simulink model "wlan_phy_tx_pmd"  (Simulink 7.8)
settings: Solver=VariableStepDiscrete  SolverMode=SingleTasking  StartTime=0.0  StopTime=inf  RelTol=1e-3
PostLoadFcn:
  | wlan_phy_tx_init
InitFcn:
  | wlan_phy_tx_init
StartFcn:
  | wlan_phy_tx_init
undefined symbols (not defined in the file): gcbh, ht_preamble_rom, MAX_CP_LEN, MAX_DATA_BITS_PER_SYM_PERIOD, MAX_NCBPS, MAX_NUM_BYTES, MAX_NUM_SC, MAX_NUM_SYMS, mcs_rom_11ag, mcs_rom_11n, Mod_Constellation_16QAM, Mod_Constellation_64QAM, Mod_Constellation_BPSK, Mod_Constellation_QPSK, Preamble_IQ, Preamble_IQ_scaled, tx_sim, wlan_tx_interleave_rom, xlBlockLoadCallback, xlGetNormalizedPeriod
libraries: xbsIndex_r4 x1358, xbsEDKLib_r4 x1
(part 3 of 10)

== system wlan_phy_tx_pmd/HT Preamble Gen ==
  Sym Cfg : Inport
  Start : Inport  Port=2
  IQ FIFO tready : Inport  Port=3
  Bus Creator : BusCreator
  Concat : xbsIndex_r4/Concat  num_inputs=2  dbl_ovrd=off  block_type=concat
  Constant9 : xbsIndex_r4/Constant  const=ceil(length(ht_preamble_rom)/2) - 1  gui_display_data_type=Fixed-point  arith_type=Unsigned  n_bits=ceil(log2(length(ht_preamble_rom)))-1  bin_pt=0  preci_type=Single  exp_width=8  frac_width=24  explicit_period=off  period=1  equ=P=C  opselect=C  inp2=PCIN>>17  opr=+  inp1=P  carry=CIN  dbl_ovrd=off  block_type=constant
  Counter1 : xbsIndex_r4/Counter  cnt_type=Free Running  cnt_to=Inf  operation=Up  start_count=0  cnt_by_val=1  arith_type=Unsigned  n_bits=ceil(log2(length(ht_preamble_rom)))-1  bin_pt=0  load_pin=off  rst=on  en=on  explicit_period=off  period=1  dbl_ovrd=off  use_behavioral_HDL=off  implementation=Fabric  block_type=counter
  Delay{,1..3} (4 alike) : xbsIndex_r4/Delay  rst=off  infoeditControl=Selection of Reset will increase slice count due to use of real FFs and instead of SRLs  en=off  latency=1  dbl_ovrd=off  reg_retiming=off  block_type=delay
  HT Training I : xbsIndex_r4/ROM  depth=length(ht_preamble_rom)  initVector=real(ht_preamble_rom)  distributed_mem=Distributed memory  rst=off  init_reg=0  en=off  latency=1  gui_display_data_type=Fixed-point  arith_type="Signed  (2's comp)"  n_bits=16  bin_pt=15  preci_type=Single  exp_width=8  frac_width=24  dbl_ovrd=off  optimize=Area  use_rpm=on  block_type=sprom
  HT Training Q : xbsIndex_r4/ROM  depth=length(ht_preamble_rom)  initVector=imag(ht_preamble_rom)  distributed_mem=Distributed memory  rst=off  init_reg=0  en=off  latency=1  gui_display_data_type=Fixed-point  arith_type="Signed  (2's comp)"  n_bits=16  bin_pt=15  preci_type=Single  exp_width=8  frac_width=24  dbl_ovrd=off  optimize=Area  use_rpm=on  block_type=sprom
  Inverter1 : xbsIndex_r4/Inverter  en=off  latency=0  dbl_ovrd=off  block_type=inv
      settings: xl_area=[0 0 0 0 0 0 0]  block_version=VER_STRING_GOES_HERE
  Logical1 : xbsIndex_r4/Logical  logical_function=OR  inputs=2  en=off  latency=0  precision=Full  arith_type=Unsigned  n_bits=8  bin_pt=2  align_bp=on  dbl_ovrd=off  block_type=logical
      settings: xl_area=[1 0 0 1 0 0 0]  block_version=VER_STRING_GOES_HERE
  Logical2 : xbsIndex_r4/Logical  logical_function=OR  inputs=2  en=off  latency=0  precision=Full  arith_type=Unsigned  n_bits=8  bin_pt=2  align_bp=on  dbl_ovrd=off  block_type=logical
      settings: xl_area=[1 0 0 1 0 0 0]  block_version=VER_STRING_GOES_HERE
  Logical3 : xbsIndex_r4/Logical  logical_function=AND  inputs=2  en=off  latency=0  precision=Full  arith_type=Unsigned  n_bits=8  bin_pt=2  align_bp=on  dbl_ovrd=off  block_type=logical
      settings: xl_area=[1 0 0 1 0 0 0]  block_version=VER_STRING_GOES_HERE
  Logical4 : xbsIndex_r4/Logical  logical_function=AND  inputs=2  en=off  latency=0  precision=Full  arith_type=Unsigned  n_bits=8  bin_pt=2  align_bp=on  dbl_ovrd=off  block_type=logical
      settings: xl_area=[1 0 0 1 0 0 0]  block_version=VER_STRING_GOES_HERE
  MCode : xbsIndex_r4/MCode  mfname=sym_config_decode  explicit_period=on  period=1  inputsTable={'boundInpExpr'=>[''],'inputs'=>['sym_cfg']}  outputsTable={'outputs'=>['load_base_rate','rotate_bpsk','load_htstf','load_htltf','load_full_rate','pilot_shift','cyclic_prefix','cyclic_shift'],'suppressOut'=>['off','off','off','off','off','off','off','off']}  dbl_ovrd=off  enable_stdout=off  enable_debug=off  suppress_output=on  defparams={}  hide_port_list={}  block_type=mcode
  Relational2 : xbsIndex_r4/Relational  mode=a>=b  en=off  latency=0  dbl_ovrd=off  block_type=relational
  S-R Latch1 : Subsystem
  " Sym Cfg" : Outport
  IQ stream : Outport  Port=2
  wires:
  Counter1/1 -> Concat/2, Relational2/1
  Constant9/1 -> Relational2/2
  Inverter1/1 -> Counter1/1
  S-R Latch1/1(Q) -> Inverter1/1, Delay1/1, Logical4/1
  [TX_RESET] -> Logical2/1
  Relational2/1 -> Logical2/2, Delay2/1
  Logical2/1 -> S-R Latch1/2(R)
  Concat/1 -> HT Training I/1, HT Training Q/1
  MCode/4 -> Logical1/1, Delay3/1
  HT Training I/1 -> Bus Creator/1  "I"
  HT Training Q/1 -> Bus Creator/2  "Q"
  Logical3/1 -> S-R Latch1/1(S)
  Start/1 -> Logical3/2
  Sym Cfg/1 -> Delay/1, MCode/1
  MCode/3 -> Logical1/2
  Logical1/1 -> Logical3/1
  Delay/1 -> " Sym Cfg"/1
  Delay1/1 -> Bus Creator/3  "IQ tvalid"
  Delay2/1 -> Bus Creator/4  "IQ tlast"
  Bus Creator/1 -> IQ stream/1
  Logical4/1 -> Counter1/2
  IQ FIFO tready/1 -> Logical4/2
  Delay3/1 -> Concat/1

== system wlan_phy_tx_pmd/IFFT and Cyclic Prefix ==
  Sym Cfg : Inport
  I : Inport  Port=2
  Q : Inport  Port=3
  IQ Valid : Inport  Port=4
  IQ tlast : Inport  Port=5
  Buffer and Cyclic Prefix : Subsystem
  FFT Core : Subsystem
  FIFO : Subsystem
  " I" : Outport
  " Q" : Outport  Port=2
  " IQ Valid" : Outport  Port=3
  FIFO tready : Outport  Port=4
  wires:
  FFT Core/2(I out) -> Buffer and Cyclic Prefix/1(I)
  FFT Core/3(Q out) -> Buffer and Cyclic Prefix/2(Q)
  FFT Core/4(data_xk_index) -> Buffer and Cyclic Prefix/3(xkindex)
  FFT Core/5(data_out_tvalid) -> Buffer and Cyclic Prefix/4(tvalid)
  FFT Core/6(data_out_tlast) -> Buffer and Cyclic Prefix/5(tlast)
  FFT Core/1(data_in_tready) -> FIFO/1(FFT tready)
  FIFO/1(" I") -> FFT Core/1("I ")
  Buffer and Cyclic Prefix/1(" I") -> " I"/1
  Buffer and Cyclic Prefix/2(" Q") -> " Q"/1
  FIFO/3(" IQ tvalid") -> FFT Core/3(IQ In Valid)
  Buffer and Cyclic Prefix/3(" valid") -> " IQ Valid"/1
  FIFO/4(IQ tlast) -> FFT Core/4(IQ tlast)
  FIFO/5(Sym cfg) -> Buffer and Cyclic Prefix/6(Sym Cfg)
  Sym Cfg/1 -> FIFO/2(Sym Cfg)
  I/1 -> FIFO/3(I)
  Q/1 -> FIFO/4(Q)
  IQ Valid/1 -> FIFO/5(IQ tvalid)
  IQ tlast/1 -> FIFO/6("IQ tlast ")
  FIFO/2(" Q") -> FFT Core/2("Q ")
  FIFO/6(FIFO tready) -> FIFO tready/1

== system wlan_phy_tx_pmd/Mux ==
  Preamble Sym Cfg : Inport
  Preamble IQ : Inport  Port=2
  PSDU Sym Cfg : Inport  Port=3
  PSDU IQ : Inport  Port=4
  Bus Selector : BusSelector  OutputSignals=I,Q,IQ tvalid,IQ tlast
  Bus Selector1 : BusSelector  OutputSignals=I,Q,IQ tvalid,IQ tlast
  Mux{1..4,6} (5 alike) : xbsIndex_r4/Mux  inputs=2  en=off  latency=0  precision=Full  arith_type=Unsigned  n_bits=16  bin_pt=14  quantization=Truncate  overflow=Wrap  dbl_ovrd=off  block_type=mux
  Sym Cfg : Outport
  " I" : Outport  Port=2
  " Q" : Outport  Port=3
  " IQ tvalid" : Outport  Port=4
  IQ tlast : Outport  Port=5
  wires:
  Mux6/1 -> " I"/1
  Mux1/1 -> " Q"/1
  Mux2/1 -> " IQ tvalid"/1
  Mux3/1 -> IQ tlast/1
  Preamble IQ/1 -> Bus Selector/1
  Bus Selector/1 -> Mux6/2  "<I>"
  Bus Selector/2 -> Mux1/2  "<Q>"
  Bus Selector/3 -> Mux2/2  "<IQ tvalid>"
  Bus Selector/4 -> Mux3/2  "<IQ tlast>"
  PSDU IQ/1 -> Bus Selector1/1
  Bus Selector1/4 -> Mux3/3  "<IQ tlast>"
  Bus Selector1/1 -> Mux6/3  "<I>"
  Bus Selector1/2 -> Mux1/3  "<Q>"
  Bus Selector1/3 -> Mux2/1, Mux1/1, Mux6/1, Mux2/3, Mux3/1, Mux4/1  "<IQ tvalid>"
  PSDU Sym Cfg/1 -> Mux4/3
  Preamble Sym Cfg/1 -> Mux4/2
  Mux4/1 -> Sym Cfg/1

== system wlan_phy_tx_pmd/OFDM Symbol Ctrl ==
  note: Stop generating symbols after DATA field is complete
  note: Stop generating symbols if TX_RESET asserts early
  note: This block generates two outputs:
      | Start Sym: triggers generation of one OFDM symbol from the Tx pipeline
      | Sym Cfg: parameters required to generate the new OFDM symbol
      |
      | Timing of Start Sym is critical:
      | Immediately after "Start Tx" this block triggers computation of 3 OFDM symbols. The resulting
      | samples are stored in the FIFO in the "Outputs" block. Samples will be read from this FIFO after
      | the preamble. Once the FIFO occupancy drops below 180 samples (first 3 symbols occupy 240
      | samples), the next OFDM symbol is started. From this point forward a new OFDM symbol is
      | started every N sample periods, where N is the number of samples in the previous OFDM symbol
      | (N = num_subcarriers + cyclic_prefix_length). This timing ensures the output FIFO always has
      | enough samples to sustain a constant stream to the DACs, while adapting to changes in the
      | sampling rate and number of samples in each OFDM symbol / cyclic prefix.
      |
      | The Start Sym signal stops asserting after the final OFDM symbol is computed, indicated by the
      | DATA field being complete.
      |
      | The selection of the 180 sample threshold above is critical. A higher threshold will overflow the FIFO
      | with low MCS and low Tx sample rate. A lower thrshold will underflow the FIFO for high MCS and high
      | sample rate. This threshold will need tweaking for any big changes in Tx pipeline latency.
  Start Tx : Inport
  Sym Done : Inport  Port=2
  Data Done : Inport  Port=3
  Constant1 : xbsIndex_r4/Constant  const=180  gui_display_data_type=Fixed-point  arith_type=Unsigned  n_bits=8  bin_pt=0  preci_type=Single  exp_width=8  frac_width=24  explicit_period=off  period=1  equ=P=C  opselect=C  inp2=PCIN>>17  opr=+  inp1=P  carry=CIN  dbl_ovrd=off  block_type=constant
  Constant2 : xbsIndex_r4/Constant  const=2  gui_display_data_type=Fixed-point  arith_type=Unsigned  n_bits=2  bin_pt=0  preci_type=Single  exp_width=8  frac_width=24  explicit_period=off  period=1  equ=P=C  opselect=C  inp2=PCIN>>17  opr=+  inp1=P  carry=CIN  dbl_ovrd=off  block_type=constant
  Constant4 : xbsIndex_r4/Constant  const=20  gui_display_data_type=Fixed-point  arith_type=Unsigned  n_bits=5  bin_pt=0  preci_type=Single  exp_width=8  frac_width=24  explicit_period=off  period=1  equ=P=C  opselect=C  inp2=PCIN>>17  opr=+  inp1=P  carry=CIN  dbl_ovrd=off  block_type=constant
  Gateway Out{1..6,10} (7 alike) : xbsIndex_r4/Gateway Out  inherit_from_input=off  hdl_port=off  timing_constraint=None  locs_specified=off  LOCs={}  UseAsDAC=off  DACChannel='1'  block_type=gatewayout
  Inverter1 : xbsIndex_r4/Inverter  en=off  latency=0  dbl_ovrd=off  block_type=inv
  Inverter2 : xbsIndex_r4/Inverter  en=off  latency=0  dbl_ovrd=off  block_type=inv
  Logical1 : xbsIndex_r4/Logical  logical_function=AND  inputs=2  en=off  latency=0  precision=Full  arith_type=Unsigned  n_bits=8  bin_pt=2  align_bp=on  dbl_ovrd=off  block_type=logical
      settings: xl_area=[1 0 0 1 0 0 0]  block_version=VER_STRING_GOES_HERE
  Logical2 : xbsIndex_r4/Logical  logical_function=OR  inputs=4  en=off  latency=0  precision=Full  arith_type=Unsigned  n_bits=8  bin_pt=2  align_bp=on  dbl_ovrd=off  block_type=logical
      settings: xl_area=[1 0 0 1 0 0 0]  block_version=VER_STRING_GOES_HERE
  Logical3 : xbsIndex_r4/Logical  logical_function=AND  inputs=2  en=off  latency=0  precision=Full  arith_type=Unsigned  n_bits=8  bin_pt=2  align_bp=on  dbl_ovrd=off  block_type=logical
      settings: xl_area=[1 0 0 1 0 0 0]  block_version=VER_STRING_GOES_HERE
  Logical4 : xbsIndex_r4/Logical  logical_function=AND  inputs=3  en=off  latency=0  precision=Full  arith_type=Unsigned  n_bits=8  bin_pt=2  align_bp=on  dbl_ovrd=off  block_type=logical
      settings: xl_area=[1 0 0 1 0 0 0]  block_version=VER_STRING_GOES_HERE
  Logical5 : xbsIndex_r4/Logical  logical_function=AND  inputs=2  en=off  latency=0  precision=Full  arith_type=Unsigned  n_bits=8  bin_pt=2  align_bp=on  dbl_ovrd=off  block_type=logical
      settings: xl_area=[1 0 0 1 0 0 0]  block_version=VER_STRING_GOES_HERE
  Posedge1 : Subsystem
  Posedge2 : Subsystem
  Posedge3 : Subsystem
  Relational1 : xbsIndex_r4/Relational  mode=a<b  en=off  latency=0  dbl_ovrd=off  block_type=relational
  Relational2 : xbsIndex_r4/Relational  mode=a<=b  en=off  latency=0  dbl_ovrd=off  block_type=relational
  S-R Latch1 : Subsystem
  S-R Latch2 : Subsystem
  S-R Latch3 : Subsystem
  Slice : xbsIndex_r4/Slice  nbits=5  boolean_output=off  mode=Lower Bit Location + Width  bit1=0  base1=MSB of Input  bit0=0  base0=LSB of Input  dbl_ovrd=off  block_type=slice
  Sym Config Encode : Subsystem
  Sym Counter : Subsystem
  Sym Samp Counter : Subsystem
  Sym Start Ctrl : Scope  NumInputPorts=7
      settings: TimeRange=20000  YMin=0~0~0~0~0~0~0  YMax=1~1~1~1~250~7~16  SaveName=ScopeData3
  Sym Cfg : Outport
  " Start Sym" : Outport  Port=2
  wires:
  Sym Config Encode/1(Sym Cfg) -> Sym Cfg/1, Sym Samp Counter/2(Sym Cfg), Slice/1
  Sym Counter/1(Sym Ind) -> Relational1/1, Sym Config Encode/1(OFDM Sym Ind), Gateway Out6/1
  Gateway Out10/1 -> Sym Start Ctrl/3  "Sym Start"
  Gateway Out5/1 -> Sym Start Ctrl/4  "Sym Done"
  [OUTPUT_FIFO_OCC] -> Gateway Out1/1
  Gateway Out1/1 -> Sym Start Ctrl/5  "DAC FIFO Occ"
  Constant2/1 -> Relational1/2
  Start Tx/1 -> Posedge1/1(D)
  Sym Counter/2(" Start Sym") -> Logical4/1
  Posedge1/1(Q) -> Logical2/1, Gateway Out2/1, S-R Latch2/1(S)
  Sym Done/1 -> Gateway Out5/1, Logical3/2
  Relational1/1 -> Logical3/1
  Logical3/1 -> Logical2/2
  [OUTPUT_FIFO_OCC] -> Relational2/1
  Relational2/1 -> Posedge2/1(D)
  Constant1/1 -> Relational2/2
  Gateway Out2/1 -> Sym Start Ctrl/1  "Tx Start"
  Gateway Out3/1 -> Sym Start Ctrl/2  "Data Done"
  Gateway Out4/1 -> Sym Start Ctrl/7  "Sym Cfg"
  Gateway Out6/1 -> Sym Start Ctrl/6  "Sym Index"
  S-R Latch3/1(Q) -> Logical1/1, Inverter2/1
  Posedge3/1(Q) -> S-R Latch1/1(S), Gateway Out3/1
  Data Done/1 -> Posedge3/1(D)
  S-R Latch1/1(Q) -> Inverter1/1
  Logical4/1 -> " Start Sym"/1, Sym Samp Counter/1(Sym Started), Gateway Out10/1
  Inverter1/1 -> Logical4/2
  S-R Latch2/1(Q) -> Logical4/3
  Logical2/1 -> Sym Counter/1(Start Sym)
  Posedge2/1(Q) -> S-R Latch3/1(S), Logical5/1
  Sym Samp Counter/1(Start Next) -> Logical1/2
  Logical1/1 -> Logical2/4
  [TX_RESET] -> S-R Latch2/2(R), S-R Latch3/2(R), S-R Latch1/2(R)
  Slice/1 -> Gateway Out4/1
  Logical5/1 -> Logical2/3
  Inverter2/1 -> Logical5/2

== system wlan_phy_tx_pmd/PSDU Syms Gen ==
  note: This block implements the actual Tx PHY pipeline, from data bits to I/Q samples.
  Sym Cfg : Inport
  Start Sym : Inport  Port=2
  IQ FIFO tready : Inport  Port=3
  Bus Creator : BusCreator
  Convolutional Encoder : Subsystem
  Index Gen : Subsystem
  Modulate : Subsystem
  Pkt Data : Subsystem
  Puncture & Interleave : Subsystem
  " Sym Cfg" : Outport
  IQ stream : Outport  Port=2
  DATA Done : Outport  Port=3
  wires:
  Start Sym/1 -> Index Gen/2(Start Sym)
  Sym Cfg/1 -> Index Gen/1(Sym Cfg)
  Index Gen/1(" Sym Cfg") -> Pkt Data/1(Sym Cfg)
  Index Gen/2(Byte Ind) -> Pkt Data/2(Byte Ind)
  Index Gen/3(Byte Ind Valid) -> Pkt Data/3("Byte Ind Valid ")
  Index Gen/4(Bit Sel) -> Pkt Data/4(Bit Sel)
  Index Gen/5(Bit Sel Valid) -> Pkt Data/5(Bit Sel Valid)
  Pkt Data/1(" Sym Cfg") -> Convolutional Encoder/1(Sym Cfg)
  Pkt Data/2(Tx Bit) -> Convolutional Encoder/2(Tx Bit)
  Pkt Data/3(Tx Bit tvalid) -> Convolutional Encoder/3(Tx Bit tvalid)
  Pkt Data/5(DATA Done) -> DATA Done/1
  Pkt Data/4(Tx Bit tlast) -> Convolutional Encoder/4(Tx Bit tlast)
  Convolutional Encoder/1(" Sym Cfg") -> Puncture & Interleave/2(Sym Cfg)
  Convolutional Encoder/2(Enc Bit A) -> Puncture & Interleave/3(Bit A)
  Convolutional Encoder/3(Enc Bit B) -> Puncture & Interleave/4(Bit B)
  Convolutional Encoder/4(Enc Bits tvalid) -> Puncture & Interleave/5(Bits tvalid)
  Convolutional Encoder/5(Enc Bits tlast) -> Puncture & Interleave/6(Bits tlast)
  Modulate/1(Data Sym Ind) -> Puncture & Interleave/1(Data Sym Ind)
  Puncture & Interleave/2(Sc Bits) -> Modulate/2(Sc Bits)
  Puncture & Interleave/1(" Sym Cfg") -> Modulate/1(Sym Cfg)
  Puncture & Interleave/3(Sym Bits Rdy) -> Modulate/3(Sym Bits Rdy)
  Modulate/3(I) -> Bus Creator/1  "I"
  Modulate/4(Q) -> Bus Creator/2  "Q"
  Bus Creator/1 -> IQ stream/1
  Modulate/5(IQ tvalid) -> Bus Creator/3  "IQ tvalid"
  Modulate/6(IQ tlast) -> Bus Creator/4  "IQ tlast"
  Modulate/2(" Sym Cfg") -> " Sym Cfg"/1
  IQ FIFO tready/1 -> Modulate/4(IQ FIFO tready)

== system wlan_phy_tx_pmd/Preamble & Outputs ==
  note: 1 sample period + margin
      | for ctrl latencies
  note: DFFs to isolate FIFO inputs from combinational
      | signals, part of the hardware/sim mismatch debug.
      | See note in FIFO block for more info.
  Tx Start : Inport
  I : Inport  Port=2
  Q : Inport  Port=3
  IQ tvalid : Inport  Port=4
  DAC Outputs : Subsystem
  Delay2 : xbsIndex_r4/Delay  rst=off  infoeditControl=Selection of Reset will increase slice count due to use of real FFs and instead of SRLs  en=off  latency=12  dbl_ovrd=off  reg_retiming=off  block_type=delay
  End of Tx Ctrl : Subsystem
  FIFO : Subsystem
  Gateway Out{1..3,6,14} (5 alike) : xbsIndex_r4/Gateway Out  inherit_from_input=off  hdl_port=off  timing_constraint=None  locs_specified=off  LOCs={}  UseAsDAC=off  DACChannel='1'  block_type=gatewayout
  Logical2 : xbsIndex_r4/Logical  logical_function=AND  inputs=3  en=off  latency=0  precision=Full  arith_type=Unsigned  n_bits=16  bin_pt=0  align_bp=on  dbl_ovrd=off  block_type=logical
  Logical3 : xbsIndex_r4/Logical  logical_function=AND  inputs=2  en=off  latency=0  precision=Full  arith_type=Unsigned  n_bits=16  bin_pt=0  align_bp=on  dbl_ovrd=off  block_type=logical
  Outputs : Scope  NumInputPorts=10
      settings: TimeRange=6000  YMin=0~0~0~0~-1~-1~-0.1~-1~-0.5~-1  YMax=1~1~250~1~1~1~1.1~0.5~0.5~1  SaveName=ScopeData20
  Posedge : Subsystem
  Preamble Gen : Subsystem
  Real-Imag to Complex : RealImagToComplex
  Register2 : xbsIndex_r4/Register  init=0  rst=off  en=off  dbl_ovrd=off  block_type=register
  Register3 : xbsIndex_r4/Register  init=0  rst=off  en=off  dbl_ovrd=off  block_type=register
  Register4 : xbsIndex_r4/Register  init=0  rst=off  en=off  dbl_ovrd=off  block_type=register
  S-R Latch : Subsystem
  Scaling : Subsystem
  To Workspace : ToWorkspace  VariableName=wlan_tx_out  SampleTime=-1  SaveFormat=Array
      settings: Decimation=160 / tx_sim.samp_rate
  tag scope: LAST_SAMP_OUTPUT_TO_DACS=global
  wires:
  Logical2/1 -> Register3/1, Register4/1
  Posedge/1(Q) -> S-R Latch/1(S), FIFO/1(Reset)
  Tx Start/1 -> Posedge/1(D), Gateway Out14/1
  [TX_RESET] -> S-R Latch/2(R)
  S-R Latch/1(Q) -> Preamble Gen/1(Tx Running), Logical2/2, End of Tx Ctrl/2(Tx Started)
  Q/1 -> FIFO/3(FFT Q)
  IQ tvalid/1 -> FIFO/4(Write), Gateway Out6/1
  FIFO/1(" I") -> Scaling/4(Payload I)
  DAC Outputs/1(" I") -> Real-Imag to Complex/1, Outputs/8  "DAC I"
  Preamble Gen/2(I) -> Scaling/2(Preamble I)
  Gateway Out14/1 -> Outputs/1  "Tx Start"
  Gateway Out1/1 -> Outputs/2  "Preamble Done"
  Gateway Out2/1 -> Outputs/3  "FIFO Occ"
  Gateway Out3/1 -> Outputs/4  "FIFO Rd En"
  Preamble Gen/1(Done) -> Gateway Out1/1, Scaling/1(Payload Sel)
  Real-Imag to Complex/1 -> To Workspace/1
  DAC Outputs/2(" Q") -> Real-Imag to Complex/2, Outputs/9  "DAC Q"
  Preamble Gen/3(Q) -> Scaling/3(Preamble Q)
  FIFO/2(" Q") -> Scaling/5(Payload Q)
  Scaling/1(" I") -> DAC Outputs/1(I)
  Gateway Out6/1 -> Outputs/7  "FIFO Wr En"
  Preamble Gen/4(Early Done) -> Logical2/1
  I/1 -> FIFO/2(FFT I)
  FIFO/3(" Empty") -> Logical3/1, End of Tx Ctrl/1(FIFO Emtpy)
  [TX_IQ_SAMP_CE] -> Logical2/3, Register2/1
  End of Tx Ctrl/1(Output En) -> DAC Outputs/3(En)
  Logical3/1 -> Delay2/1
  Delay2/1 -> [LAST_SAMP_OUTPUT_TO_DACS]
  Register2/1 -> Preamble Gen/2(Rd En)
  Register3/1 -> FIFO/5(Rd), Gateway Out3/1
  Register4/1 -> Logical3/2
  [OUTPUT_FIFO_OCC] -> Gateway Out2/1
  Scaling/2(" Q") -> DAC Outputs/2(Q)

== system wlan_phy_tx_pmd/Radio Controller & MAC IO ==
  note: MAC I/O
  note: Radio Controller I/O
  note: Mimic hardware delay between MAC start and RC start
  Constant : Constant  Value=0
  Constant1 : Constant
  Constant3 : Constant  Value=tx_sim.PHY_mode
  Convert1 : xbsIndex_r4/Convert  gui_display_data_type=Boolean  arith_type=Boolean  n_bits=1  bin_pt=0  float_type=Single  exp_bits=8  fraction_bits=24  quantization=Truncate  overflow=Wrap  en=off  latency=0  dbl_ovrd=off  pipeline=off  block_type=convert
  Convert2 : xbsIndex_r4/Convert  gui_display_data_type=Boolean  arith_type=Boolean  n_bits=1  bin_pt=0  float_type=Single  exp_bits=8  fraction_bits=24  quantization=Truncate  overflow=Wrap  en=off  latency=0  dbl_ovrd=off  pipeline=off  block_type=convert
  Delay : Delay  DelayLength=16
  Logical Operator : Logic  Operator=OR  AllPortsSameDT=off  OutDataTypeStr=boolean
  PHY_TX_ANT_MASK : xbsIndex_r4/Gateway In  gui_display_data_type=Fixed-point  arith_type=Unsigned  n_bits=4  bin_pt=0  preci_type=Single  exp_width=8  frac_width=24  quantization="Round  (unbiased: +/- Inf)"  overflow=Saturate  period=1  dbl_ovrd=off  timing_constraint=None  locs_specified=off  LOCs={}  UseAsADC=off  ADCChannel='1'  inherit_from_input=off  hdl_port=on  block_type=gatewayin
  PHY_TX_DONE : xbsIndex_r4/Gateway Out  inherit_from_input=off  hdl_port=on  timing_constraint=None  locs_specified=off  LOCs={}  UseAsDAC=off  DACChannel='1'  block_type=gatewayout
  PHY_TX_PHY_MODE : xbsIndex_r4/Gateway In  gui_display_data_type=Fixed-point  arith_type=Unsigned  n_bits=3  bin_pt=0  preci_type=Single  exp_width=8  frac_width=24  quantization="Round  (unbiased: +/- Inf)"  overflow=Saturate  period=1  dbl_ovrd=off  timing_constraint=None  locs_specified=off  LOCs={}  UseAsADC=off  ADCChannel='1'  inherit_from_input=off  hdl_port=on  block_type=gatewayin
  PHY_TX_PKT_BUF : xbsIndex_r4/Gateway In  gui_display_data_type=Fixed-point  arith_type=Unsigned  n_bits=4  bin_pt=0  preci_type=Single  exp_width=8  frac_width=24  quantization="Round  (unbiased: +/- Inf)"  overflow=Saturate  period=1  dbl_ovrd=off  timing_constraint=None  locs_specified=off  LOCs={}  UseAsADC=off  ADCChannel='1'  inherit_from_input=off  hdl_port=on  block_type=gatewayin
  PHY_TX_START : xbsIndex_r4/Gateway In  gui_display_data_type=Fixed-point  arith_type=Unsigned  n_bits=1  bin_pt=0  preci_type=Single  exp_width=8  frac_width=24  quantization="Round  (unbiased: +/- Inf)"  overflow=Saturate  period=1  dbl_ovrd=off  timing_constraint=None  locs_specified=off  LOCs={}  UseAsADC=off  ADCChannel='1'  inherit_from_input=off  hdl_port=on  block_type=gatewayin
  PHY_TX_STARTED : xbsIndex_r4/Gateway Out  inherit_from_input=off  hdl_port=on  timing_constraint=None  locs_specified=off  LOCs={}  UseAsDAC=off  DACChannel='1'  block_type=gatewayout
  Pulse Generator1 : DiscretePulseGenerator  Period=1e9  PulseWidth=100  PhaseDelay=150
  RC_PHY_START : xbsIndex_r4/Gateway In  gui_display_data_type=Fixed-point  arith_type=Unsigned  n_bits=1  bin_pt=0  preci_type=Single  exp_width=8  frac_width=24  quantization="Round  (unbiased: +/- Inf)"  overflow=Saturate  period=1  dbl_ovrd=off  timing_constraint=None  locs_specified=off  LOCs={}  UseAsADC=off  ADCChannel='1'  inherit_from_input=off  hdl_port=on  block_type=gatewayin
  RC_TX_GAIN_A : xbsIndex_r4/Gateway Out  inherit_from_input=off  hdl_port=on  timing_constraint=None  locs_specified=off  LOCs={}  UseAsDAC=off  DACChannel='1'  block_type=gatewayout
  RC_TX_GAIN_B : xbsIndex_r4/Gateway Out  inherit_from_input=off  hdl_port=on  timing_constraint=None  locs_specified=off  LOCs={}  UseAsDAC=off  DACChannel='1'  block_type=gatewayout
  RC_TX_GAIN_C : xbsIndex_r4/Gateway Out  inherit_from_input=off  hdl_port=on  timing_constraint=None  locs_specified=off  LOCs={}  UseAsDAC=off  DACChannel='1'  block_type=gatewayout
  RC_TX_GAIN_D : xbsIndex_r4/Gateway Out  inherit_from_input=off  hdl_port=on  timing_constraint=None  locs_specified=off  LOCs={}  UseAsDAC=off  DACChannel='1'  block_type=gatewayout
  RC_USR_RXEN : xbsIndex_r4/Gateway Out  inherit_from_input=off  hdl_port=on  timing_constraint=None  locs_specified=off  LOCs={}  UseAsDAC=off  DACChannel='1'  block_type=gatewayout
  RC_USR_TXEN_A : xbsIndex_r4/Gateway Out  inherit_from_input=off  hdl_port=on  timing_constraint=None  locs_specified=off  LOCs={}  UseAsDAC=off  DACChannel='1'  block_type=gatewayout
  RC_USR_TXEN_B : xbsIndex_r4/Gateway Out  inherit_from_input=off  hdl_port=on  timing_constraint=None  locs_specified=off  LOCs={}  UseAsDAC=off  DACChannel='1'  block_type=gatewayout
  RC_USR_TXEN_C : xbsIndex_r4/Gateway Out  inherit_from_input=off  hdl_port=on  timing_constraint=None  locs_specified=off  LOCs={}  UseAsDAC=off  DACChannel='1'  block_type=gatewayout
  RC_USR_TXEN_D : xbsIndex_r4/Gateway Out  inherit_from_input=off  hdl_port=on  timing_constraint=None  locs_specified=off  LOCs={}  UseAsDAC=off  DACChannel='1'  block_type=gatewayout
  tag scope: MAC_IO_PHY_TX_ANT_MASK=global, MAC_IO_PHY_TX_PHY_MODE=global, MAC_IO_PHY_TX_PKT_BUF=global, MAC_IO_PHY_TX_START=global, RC_IO_PHY_START=global
  wires:
  PHY_TX_START/1 -> Convert1/1
  PHY_TX_ANT_MASK/1 -> [MAC_IO_PHY_TX_ANT_MASK]
  PHY_TX_PKT_BUF/1 -> [MAC_IO_PHY_TX_PKT_BUF]
  [MAC_IO_PHY_TX_STARTED] -> PHY_TX_STARTED/1
  [MAC_IO_PHY_TX_DONE] -> PHY_TX_DONE/1
  Constant/1 -> PHY_TX_PKT_BUF/1
  Constant1/1 -> PHY_TX_ANT_MASK/1
  [RC_IO_TXEN_A] -> RC_USR_TXEN_A/1
  [RC_IO_TXEN_D] -> RC_USR_TXEN_D/1
  [RC_IO_TXEN_C] -> RC_USR_TXEN_C/1
  [RC_IO_TXEN_B] -> RC_USR_TXEN_B/1
  [RC_IO_RXEN] -> RC_USR_RXEN/1
  [RC_IO_TX_GAIN_A] -> RC_TX_GAIN_A/1
  [RC_IO_TX_GAIN_B] -> RC_TX_GAIN_B/1
  [RC_IO_TX_GAIN_C] -> RC_TX_GAIN_C/1
  [RC_IO_TX_GAIN_D] -> RC_TX_GAIN_D/1
  Convert1/1 -> [MAC_IO_PHY_TX_START]
  Convert2/1 -> [RC_IO_PHY_START]
  Constant3/1 -> PHY_TX_PHY_MODE/1
  PHY_TX_PHY_MODE/1 -> [MAC_IO_PHY_TX_PHY_MODE]
  Logical Operator/1 -> PHY_TX_START/1, Delay/1
  Delay/1 -> RC_PHY_START/1
  Pulse Generator1/1 -> Logical Operator/1
  [sim_Start_New_Tx] -> Logical Operator/2
  RC_PHY_START/1 -> Convert2/1

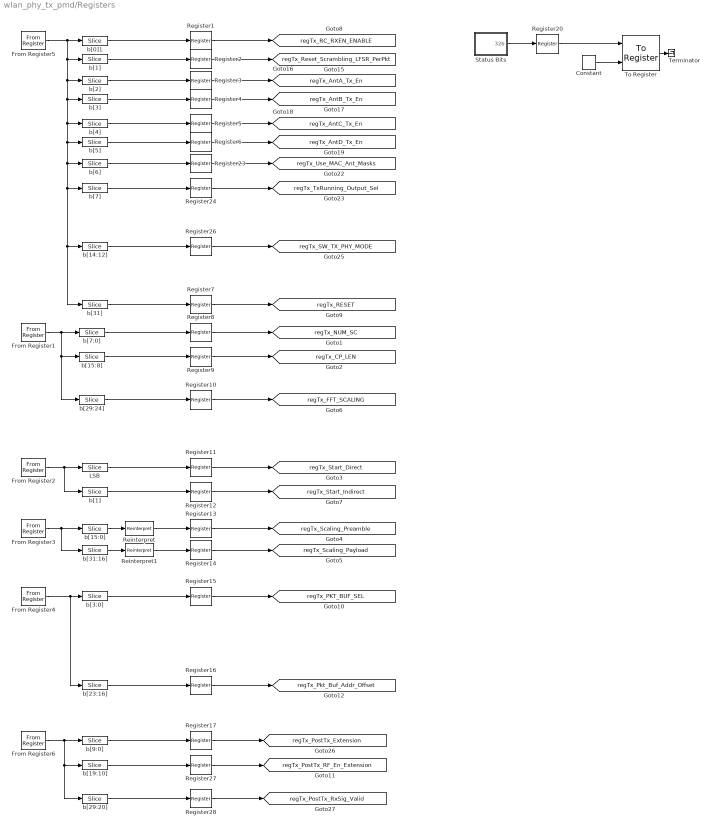
== system wlan_phy_tx_pmd/Registers ==
  Constant : xbsIndex_r4/Constant  const=1  gui_display_data_type=Boolean  arith_type=Boolean  n_bits=16  bin_pt=14  preci_type=Single  exp_width=8  frac_width=24  explicit_period=on  period=1  equ=P=C  opselect=C  inp2=PCIN>>17  opr=+  inp1=P  carry=CIN  dbl_ovrd=off  block_type=constant
  From Register1 : xbsIndex_r4/From Register  shared_memory_name='FFT_Config'  init=REG_TX_FFT_Config  period=1  ownership=Locally owned and initialized  gui_display_data_type=Fixed-point  arith_type=Unsigned  n_bits=32  bin_pt=0  preci_type=Single  dbl_ovrd=off  block_type=fromreg
      settings: AttributesFormatString=<< %<shared_memory_name> >>  infoedit="Register block that reads data to a shared memory register.  Delay of one sample period."
  From Register2 : xbsIndex_r4/From Register  shared_memory_name='TX_START'  init=0  period=1  ownership=Locally owned and initialized  gui_display_data_type=Fixed-point  arith_type=Unsigned  n_bits=32  bin_pt=0  preci_type=Single  dbl_ovrd=off  block_type=fromreg
      settings: AttributesFormatString=<< %<shared_memory_name> >>  infoedit="Register block that reads data to a shared memory register.  Delay of one sample period."
  From Register3 : xbsIndex_r4/From Register  shared_memory_name='Output_Scaling'  init=REG_TX_Output_Scaling  period=1  ownership=Locally owned and initialized  gui_display_data_type=Fixed-point  arith_type=Unsigned  n_bits=32  bin_pt=0  preci_type=Single  dbl_ovrd=off  block_type=fromreg
      settings: AttributesFormatString=<< %<shared_memory_name> >>  infoedit="Register block that reads data to a shared memory register.  Delay of one sample period."
  From Register4 : xbsIndex_r4/From Register  shared_memory_name='PKT_BUF_SEL'  init=REG_TX_PKT_BUF_SEL  period=1  ownership=Locally owned and initialized  gui_display_data_type=Fixed-point  arith_type=Unsigned  n_bits=32  bin_pt=0  preci_type=Single  dbl_ovrd=off  block_type=fromreg
      settings: AttributesFormatString=<< %<shared_memory_name> >>  infoedit="Register block that reads data to a shared memory register.  Delay of one sample period."
  From Register5 : xbsIndex_r4/From Register  shared_memory_name='Config'  init=REG_TX_Config  period=1  ownership=Locally owned and initialized  gui_display_data_type=Fixed-point  arith_type=Unsigned  n_bits=32  bin_pt=0  preci_type=Single  dbl_ovrd=off  block_type=fromreg
      settings: AttributesFormatString=<< %<shared_memory_name> >>  infoedit="Register block that reads data to a shared memory register.  Delay of one sample period."
  From Register6 : xbsIndex_r4/From Register  shared_memory_name='Timing'  init=REG_Tx_Timing  period=1  ownership=Locally owned and initialized  gui_display_data_type=Fixed-point  arith_type=Unsigned  n_bits=32  bin_pt=0  preci_type=Single  dbl_ovrd=off  block_type=fromreg
      settings: AttributesFormatString=<< %<shared_memory_name> >>  infoedit="Register block that reads data to a shared memory register.  Delay of one sample period."
  LSB : xbsIndex_r4/Slice  nbits=1  boolean_output=on  mode=Lower Bit Location + Width  bit1=0  base1=MSB of Input  bit0=0  base0=LSB of Input  dbl_ovrd=off  block_type=slice
      settings: block_version=VER_STRING_GOES_HERE
  Register{1..17,20,23..24,26..28} (23 alike) : xbsIndex_r4/Register  init=0  rst=off  en=off  dbl_ovrd=off  block_type=register
  Reinterpret : xbsIndex_r4/Reinterpret  force_arith_type=on  arith_type=Unsigned  force_bin_pt=on  bin_pt=12  block_type=reinterpret
  Reinterpret1 : xbsIndex_r4/Reinterpret  force_arith_type=on  arith_type=Unsigned  force_bin_pt=on  bin_pt=12  block_type=reinterpret
  Status Bits : Subsystem
  Terminator : Terminator
  To Register : xbsIndex_r4/To Register  shared_memory_name='STATUS'  init=0  ownership=Locally owned and initialized  explicit_data_type=on  gui_display_data_type=Fixed-point  arith_type=Unsigned  n_bits=32  bin_pt=0  preci_type=Single  dbl_ovrd=off  block_type=toreg
      settings: AttributesFormatString=<< %<shared_memory_name> >>  infoedit="Register block that writes data to a shared memory register.  Delay of one sample period."
  b[0]1 : xbsIndex_r4/Slice  nbits=1  boolean_output=on  mode=Lower Bit Location + Width  bit1=0  base1=MSB of Input  bit0=0  base0=LSB of Input  dbl_ovrd=off  block_type=slice
      settings: block_version=VER_STRING_GOES_HERE
  b[14:12] : xbsIndex_r4/Slice  nbits=3  boolean_output=off  mode=Lower Bit Location + Width  bit1=0  base1=MSB of Input  bit0=12  base0=LSB of Input  dbl_ovrd=off  block_type=slice
      settings: block_version=VER_STRING_GOES_HERE
  b[15:0] : xbsIndex_r4/Slice  nbits=16  boolean_output=off  mode=Lower Bit Location + Width  bit1=0  base1=MSB of Input  bit0=0  base0=LSB of Input  dbl_ovrd=off  block_type=slice
      settings: block_version=VER_STRING_GOES_HERE
  b[15:8] : xbsIndex_r4/Slice  nbits=8  boolean_output=off  mode=Lower Bit Location + Width  bit1=0  base1=MSB of Input  bit0=8  base0=LSB of Input  dbl_ovrd=off  block_type=slice
      settings: block_version=VER_STRING_GOES_HERE
  b[19:10] : xbsIndex_r4/Slice  nbits=10  boolean_output=off  mode=Lower Bit Location + Width  bit1=0  base1=MSB of Input  bit0=10  base0=LSB of Input  dbl_ovrd=off  block_type=slice
      settings: block_version=VER_STRING_GOES_HERE
  b[1] : xbsIndex_r4/Slice  nbits=1  boolean_output=on  mode=Lower Bit Location + Width  bit1=0  base1=MSB of Input  bit0=1  base0=LSB of Input  dbl_ovrd=off  block_type=slice
      settings: block_version=VER_STRING_GOES_HERE
  "b[1]  " : xbsIndex_r4/Slice  nbits=1  boolean_output=on  mode=Lower Bit Location + Width  bit1=0  base1=MSB of Input  bit0=1  base0=LSB of Input  dbl_ovrd=off  block_type=slice
      settings: block_version=VER_STRING_GOES_HERE
  "b[23:16] " : xbsIndex_r4/Slice  nbits=8  boolean_output=off  mode=Lower Bit Location + Width  bit1=0  base1=MSB of Input  bit0=16  base0=LSB of Input  dbl_ovrd=off  block_type=slice
      settings: block_version=VER_STRING_GOES_HERE
  b[29:20] : xbsIndex_r4/Slice  nbits=10  boolean_output=off  mode=Lower Bit Location + Width  bit1=0  base1=MSB of Input  bit0=20  base0=LSB of Input  dbl_ovrd=off  block_type=slice
      settings: block_version=VER_STRING_GOES_HERE
  b[29:24] : xbsIndex_r4/Slice  nbits=6  boolean_output=off  mode=Lower Bit Location + Width  bit1=0  base1=MSB of Input  bit0=24  base0=LSB of Input  dbl_ovrd=off  block_type=slice
      settings: block_version=VER_STRING_GOES_HERE
  b[2] : xbsIndex_r4/Slice  nbits=1  boolean_output=on  mode=Lower Bit Location + Width  bit1=0  base1=MSB of Input  bit0=2  base0=LSB of Input  dbl_ovrd=off  block_type=slice
      settings: block_version=VER_STRING_GOES_HERE
  b[31:16] : xbsIndex_r4/Slice  nbits=16  boolean_output=off  mode=Lower Bit Location + Width  bit1=0  base1=MSB of Input  bit0=16  base0=LSB of Input  dbl_ovrd=off  block_type=slice
      settings: block_version=VER_STRING_GOES_HERE
  b[31] : xbsIndex_r4/Slice  nbits=1  boolean_output=off  mode=Lower Bit Location + Width  bit1=0  base1=MSB of Input  bit0=31  base0=LSB of Input  dbl_ovrd=off  block_type=slice
      settings: block_version=VER_STRING_GOES_HERE
  b[3:0] : xbsIndex_r4/Slice  nbits=4  boolean_output=off  mode=Lower Bit Location + Width  bit1=0  base1=MSB of Input  bit0=0  base0=LSB of Input  dbl_ovrd=off  block_type=slice
      settings: block_version=VER_STRING_GOES_HERE
  b[3] : xbsIndex_r4/Slice  nbits=1  boolean_output=on  mode=Lower Bit Location + Width  bit1=0  base1=MSB of Input  bit0=3  base0=LSB of Input  dbl_ovrd=off  block_type=slice
      settings: block_version=VER_STRING_GOES_HERE
  b[4] : xbsIndex_r4/Slice  nbits=1  boolean_output=on  mode=Lower Bit Location + Width  bit1=0  base1=MSB of Input  bit0=4  base0=LSB of Input  dbl_ovrd=off  block_type=slice
      settings: block_version=VER_STRING_GOES_HERE
  b[5] : xbsIndex_r4/Slice  nbits=1  boolean_output=on  mode=Lower Bit Location + Width  bit1=0  base1=MSB of Input  bit0=5  base0=LSB of Input  dbl_ovrd=off  block_type=slice
      settings: block_version=VER_STRING_GOES_HERE
  b[6] : xbsIndex_r4/Slice  nbits=1  boolean_output=on  mode=Lower Bit Location + Width  bit1=0  base1=MSB of Input  bit0=6  base0=LSB of Input  dbl_ovrd=off  block_type=slice
      settings: block_version=VER_STRING_GOES_HERE
  b[7:0] : xbsIndex_r4/Slice  nbits=8  boolean_output=off  mode=Lower Bit Location + Width  bit1=0  base1=MSB of Input  bit0=0  base0=LSB of Input  dbl_ovrd=off  block_type=slice
      settings: block_version=VER_STRING_GOES_HERE
  b[7] : xbsIndex_r4/Slice  nbits=1  boolean_output=on  mode=Lower Bit Location + Width  bit1=0  base1=MSB of Input  bit0=7  base0=LSB of Input  dbl_ovrd=off  block_type=slice
      settings: block_version=VER_STRING_GOES_HERE
  b[9:0] : xbsIndex_r4/Slice  nbits=10  boolean_output=off  mode=Lower Bit Location + Width  bit1=0  base1=MSB of Input  bit0=0  base0=LSB of Input  dbl_ovrd=off  block_type=slice
      settings: block_version=VER_STRING_GOES_HERE
  tag scope: regTx_AntA_Tx_En=global, regTx_AntB_Tx_En=global, regTx_AntC_Tx_En=global, regTx_AntD_Tx_En=global, regTx_CP_LEN=global, regTx_FFT_SCALING=global, regTx_NUM_SC=global, regTx_PKT_BUF_SEL=global, regTx_Pkt_Buf_Addr_Offset=global, regTx_PostTx_Extension=global, regTx_PostTx_RF_En_Extension=global, regTx_PostTx_RxSig_Valid=global, regTx_RC_RXEN_ENABLE=global, regTx_RESET=global, regTx_Reset_Scrambling_LFSR_PerPkt=global, regTx_SW_TX_PHY_MODE=global, regTx_Scaling_Payload=global, regTx_Scaling_Preamble=global, regTx_Start_Direct=global, regTx_Start_Indirect=global, regTx_TxRunning_Output_Sel=global, regTx_Use_MAC_Ant_Masks=global
  wires:
  From Register5/1 -> b[0]1/1, b[1]/1, b[2]/1, b[3]/1, b[4]/1, b[5]/1, b[6]/1, b[7]/1, b[31]/1, b[14:12]/1
  From Register1/1 -> b[7:0]/1, b[15:8]/1, b[29:24]/1
  b[7:0]/1 -> Register8/1
  b[15:8]/1 -> Register9/1
  b[29:24]/1 -> Register10/1
  From Register2/1 -> LSB/1, "b[1]  "/1
  LSB/1 -> Register11/1
  From Register3/1 -> b[15:0]/1, b[31:16]/1
  b[15:0]/1 -> Reinterpret/1
  b[31:16]/1 -> Reinterpret1/1
  Reinterpret/1 -> Register13/1
  Reinterpret1/1 -> Register14/1
  "b[1]  "/1 -> Register12/1
  b[0]1/1 -> Register1/1
  b[31]/1 -> Register7/1
  Constant/1 -> To Register/2
  Status Bits/1(32b) -> Register20/1
  To Register/1 -> Terminator/1
  From Register4/1 -> b[3:0]/1, "b[23:16] "/1
  b[3:0]/1 -> Register15/1
  "b[23:16] "/1 -> Register16/1
  From Register6/1 -> b[29:20]/1, b[19:10]/1, b[9:0]/1
  b[1]/1 -> Register2/1
  b[2]/1 -> Register3/1
  b[3]/1 -> Register4/1
  b[4]/1 -> Register5/1
  b[5]/1 -> Register6/1
  Register1/1 -> [regTx_RC_RXEN_ENABLE]
  Register2/1 -> [regTx_Reset_Scrambling_LFSR_PerPkt]
  Register3/1 -> [regTx_AntA_Tx_En]
  Register4/1 -> [regTx_AntB_Tx_En]
  Register5/1 -> [regTx_AntC_Tx_En]
  Register6/1 -> [regTx_AntD_Tx_En]
  Register7/1 -> [regTx_RESET]
  Register8/1 -> [regTx_NUM_SC]
  Register9/1 -> [regTx_CP_LEN]
  Register10/1 -> [regTx_FFT_SCALING]
  Register11/1 -> [regTx_Start_Direct]
  Register12/1 -> [regTx_Start_Indirect]
  Register13/1 -> [regTx_Scaling_Preamble]
  Register14/1 -> [regTx_Scaling_Payload]
  Register15/1 -> [regTx_PKT_BUF_SEL]
  Register16/1 -> [regTx_Pkt_Buf_Addr_Offset]
  Register20/1 -> To Register/1
  b[6]/1 -> Register23/1
  Register23/1 -> [regTx_Use_MAC_Ant_Masks]
  b[7]/1 -> Register24/1
  Register24/1 -> [regTx_TxRunning_Output_Sel]
  b[14:12]/1 -> Register26/1
  Register26/1 -> [regTx_SW_TX_PHY_MODE]
  b[9:0]/1 -> Register17/1
  b[19:10]/1 -> Register27/1
  b[29:20]/1 -> Register28/1
  Register17/1 -> [regTx_PostTx_Extension]
  Register27/1 -> [regTx_PostTx_RF_En_Extension]
  Register28/1 -> [regTx_PostTx_RxSig_Valid]

== system wlan_phy_tx_pmd/Resets ==
  Constant : xbsIndex_r4/Constant  const=0  gui_display_data_type=Boolean  arith_type=Boolean  n_bits=16  bin_pt=14  preci_type=Single  exp_width=8  frac_width=24  explicit_period=on  period=1  equ=P=C  opselect=C  inp2=PCIN>>17  opr=+  inp1=P  carry=CIN  dbl_ovrd=off  block_type=constant
  Convert1 : xbsIndex_r4/Convert  gui_display_data_type=Boolean  arith_type=Boolean  n_bits=16  bin_pt=14  float_type=Single  exp_bits=8  fraction_bits=24  quantization=Truncate  overflow=Wrap  en=off  latency=0  dbl_ovrd=off  pipeline=off  block_type=convert
  Delay : xbsIndex_r4/Delay  rst=off  infoeditControl=Selection of Reset will increase slice count due to use of real FFs and instead of SRLs  en=off  latency=16  dbl_ovrd=off  reg_retiming=off  block_type=delay
  Gateway Out{1..4} (4 alike) : xbsIndex_r4/Gateway Out  inherit_from_input=off  hdl_port=off  timing_constraint=None  locs_specified=off  LOCs={}  UseAsDAC=off  DACChannel='1'  block_type=gatewayout
  Logical : xbsIndex_r4/Logical  logical_function=OR  inputs=3  en=off  latency=0  precision=Full  arith_type=Unsigned  n_bits=16  bin_pt=0  align_bp=on  dbl_ovrd=off  block_type=logical
  Logical1 : xbsIndex_r4/Logical  logical_function=OR  inputs=2  en=off  latency=0  precision=Full  arith_type=Unsigned  n_bits=16  bin_pt=0  align_bp=on  dbl_ovrd=off  block_type=logical
  Posedge1 : Subsystem
  Resets : Scope  NumInputPorts=7
      settings: TimeRange=10000  YMin=0~0~0~-0.1~0~-0.1~-0.1  YMax=1~1~1~1.1~25~1.1~1.1  SaveName=ScopeData18
  S-R Latch : Subsystem
  Sim Reset : Subsystem
  Simulation Multiplexer : xbsIndex_r4/Simulation Multiplexer  sim_sel=1  hw_sel=2  block_type=simmux
      settings: infoedit="Distinguish input subsystems as \"simulation only\" and \"generation only\".  The input specified For Simulation will be used during Simulink simulation.  The input specified For Generation will be used during code generation.  This block will typically be used on the output of a HW Co-Simulation, Black Box, or ModelSim subsystem.<br><br>Hardware Notes: This block costs nothing."
  tag scope: TX_FORCE_RESET=global, TX_PHY_DONE=global, TX_RESET=global
  wires:
  S-R Latch/1(Q) -> Delay/1, Gateway Out2/1, Logical/3
  Logical/1 -> [TX_RESET], Gateway Out3/1
  Logical1/1 -> Posedge1/1(D)
  Delay/1 -> S-R Latch/2(R)
  Gateway Out1/1 -> Resets/2  "Last Samp Tx"
  Gateway Out2/1 -> Resets/3  "Last Samp SR"
  Gateway Out3/1 -> Resets/4  "TX_RESET"
  [regTx_RESET] -> Convert1/1
  Convert1/1 -> [TX_FORCE_RESET], Logical/2
  [LAST_SAMP_OUTPUT_TO_DACS] -> Logical1/1
  [TX_SIG_DECODE_ERROR] -> Logical1/2, Gateway Out4/1
  Posedge1/1(Q) -> Gateway Out1/1, [TX_PHY_DONE], S-R Latch/1(S)
  Simulation Multiplexer/1 -> Logical/1
  Constant/1 -> Simulation Multiplexer/2
  Sim Reset/1(Out1) -> Simulation Multiplexer/1
  Gateway Out4/1 -> Resets/7

== system wlan_phy_tx_pmd/Sampling Clock ==
  note: Core runs at 160MHz via sysgen_clk port. All synchronous elements in the core
      | are clocked by the 160MHz sysgen_clk signal. The SAMP_CE input acts as a
      | clock enable throughout the sections of the PHY that process individual samples.
      |
      | The SAMP_CE frequency may change at run time. MAC code should avoid changing
      | SAMP_CE frequency during a transmission.
      |
      | The SAMP_CE signal must:
      | * Be valid in the sysgen_clk domain
      | * Assert for exactly 1 cycle per period
      | * Have duty cycle of:
      |   (1/32): 5MSps I/Q
      |   (1/16): 10MSps I/Q
      |     (1/8): 20MSps I/Q
      |     (1/4): 40MSps I/Q
      |
      | Other duty cycles are not tested, and are not supported on WARP v3 hardware.
  Convert2 : xbsIndex_r4/Convert  gui_display_data_type=Boolean  arith_type=Boolean  n_bits=1  bin_pt=0  float_type=Single  exp_bits=8  fraction_bits=24  quantization=Truncate  overflow=Wrap  en=off  latency=0  dbl_ovrd=off  pipeline=off  block_type=convert
  Pulse Generator2 : DiscretePulseGenerator  Period=160 / tx_sim.samp_rate
  SAMP_CE : xbsIndex_r4/Gateway In  gui_display_data_type=Fixed-point  arith_type=Unsigned  n_bits=1  bin_pt=0  preci_type=Single  exp_width=8  frac_width=24  quantization="Round  (unbiased: +/- Inf)"  overflow=Saturate  period=1  dbl_ovrd=off  timing_constraint=None  locs_specified=off  LOCs={}  UseAsADC=off  ADCChannel='1'  inherit_from_input=off  hdl_port=on  block_type=gatewayin
  tag scope: TX_IQ_SAMP_CE=global
  wires:
  Pulse Generator2/1 -> SAMP_CE/1
  Convert2/1 -> [TX_IQ_SAMP_CE]
  SAMP_CE/1 -> Convert2/1

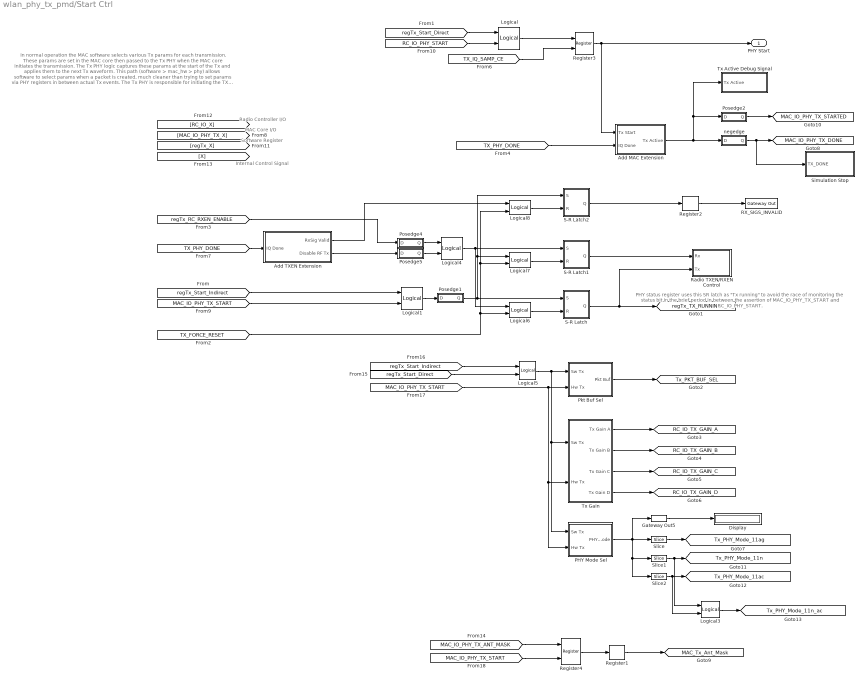
== system wlan_phy_tx_pmd/Start Ctrl ==
  note: Radio Controller I/O
  note: Software Register
  note: MAC Core I/O
  note: Internal Control Signal
  note: PHY status register uses this SR latch as "Tx running" to avoid
      | the race of monitoring the status bit in the brief period in between
      | the assertion of MAC_IO_PHY_TX_START and RC_IO_PHY_START.
  note: In normal operation the MAC software selects various Tx params for each transmission. These
      | params are set in the MAC core then passed to the Tx PHY when the MAC core initiates
      | the transmission. The Tx PHY logic captures these params at the start of the Tx and applies
      | them to the next Tx waveform. This path (software > mac_hw > phy) allows software to
      | select params when a packet is created, much cleaner than trying to set params via PHY
      | registers in between actual Tx events.
      |
      | The Tx PHY is responsible for initiating the TX mode of the radio circuit via the radio_controller
      | core. The PHY asserts the radio_controller's usr_RFx_TXEN signal. Some time later the
      | radio_controller asserts its PHY_Start ouput. This output drives the PHY's RC_PHY_START
      | input port, which begins the waveform generation pipeilne. The PHY -> RC -> PHY path
      | is indirect, but it allows good separation of hardware-dependent parameters in the RF front end
      | (sequencing of Radio/PA/PHY enables; Tx VGA gain ramp timing; etc) and the hardware-
      | independent waveform generation of the PHY.
  Add MAC Extension : Subsystem
  Add TXEN Extension : Subsystem
  Display : Display
  Gateway Out5 : xbsIndex_r4/Gateway Out  inherit_from_input=off  hdl_port=off  timing_constraint=None  locs_specified=off  LOCs={}  UseAsDAC=off  DACChannel='1'  block_type=gatewayout
  Logical{,1,3..8} (8 alike) : xbsIndex_r4/Logical  logical_function=OR  inputs=2  en=off  latency=0  precision=Full  arith_type=Unsigned  n_bits=16  bin_pt=0  align_bp=on  dbl_ovrd=off  block_type=logical
  PHY Mode Sel : Subsystem
  Pkt Buf Sel : Subsystem
  Posedge1 : Subsystem
  Posedge2 : Subsystem
  Posedge4 : Subsystem
  Posedge5 : Subsystem
  RX_SIGS_INVALID : xbsIndex_r4/Gateway Out  inherit_from_input=off  hdl_port=on  timing_constraint=None  locs_specified=off  LOCs={}  UseAsDAC=off  DACChannel='1'  block_type=gatewayout
  Radio TXEN/RXEN Control : Subsystem
  Register1 : xbsIndex_r4/Register  init=0  rst=off  en=off  dbl_ovrd=off  block_type=register
  Register2 : xbsIndex_r4/Register  init=0  rst=off  en=off  dbl_ovrd=off  block_type=register
  Register3 : xbsIndex_r4/Register  init=0  rst=off  en=on  dbl_ovrd=off  block_type=register
  Register4 : xbsIndex_r4/Register  init=0  rst=off  en=on  dbl_ovrd=off  block_type=register
      settings: xl_area=[1 1 0 0 0 0 0]  block_version=VER_STRING_GOES_HERE
  S-R Latch : Subsystem
  S-R Latch1 : Subsystem
  S-R Latch2 : Subsystem
  Simulation Stop : Subsystem
  Slice : xbsIndex_r4/Slice  nbits=1  boolean_output=on  mode=Lower Bit Location + Width  bit1=0  base1=MSB of Input  bit0=0  base0=LSB of Input  dbl_ovrd=off  block_type=slice
  Slice1 : xbsIndex_r4/Slice  nbits=1  boolean_output=on  mode=Lower Bit Location + Width  bit1=0  base1=MSB of Input  bit0=1  base0=LSB of Input  dbl_ovrd=off  block_type=slice
  Slice2 : xbsIndex_r4/Slice  nbits=1  boolean_output=on  mode=Lower Bit Location + Width  bit1=0  base1=MSB of Input  bit0=2  base0=LSB of Input  dbl_ovrd=off  block_type=slice
  Tx Active Debug Signal : Subsystem
  Tx Gain : Subsystem
  negedge : Subsystem
  PHY Start : Outport
  tag scope: MAC_IO_PHY_TX_DONE=global, MAC_IO_PHY_TX_STARTED=global, MAC_Tx_Ant_Mask=global, RC_IO_TX_GAIN_A=global, RC_IO_TX_GAIN_B=global, RC_IO_TX_GAIN_C=global, RC_IO_TX_GAIN_D=global, Tx_PHY_Mode_11ac=global, Tx_PHY_Mode_11ag=global, Tx_PHY_Mode_11n=global, Tx_PHY_Mode_11n_ac=global, Tx_PKT_BUF_SEL=global, regTx_TX_RUNNING=global
  wires:
  S-R Latch/1(Q) -> [regTx_TX_RUNNING], Radio TXEN/RXEN Control/2(Tx)
  Logical1/1 -> Posedge1/1(D)
  [MAC_IO_PHY_TX_START] -> Logical1/2
  [regTx_Start_Indirect] -> Logical1/1
  S-R Latch1/1(Q) -> Radio TXEN/RXEN Control/1(Rx)
  Logical4/1 -> S-R Latch1/1(S), Logical6/1
  Add TXEN Extension/2(Disable RF Tx) -> Posedge5/1(D)
  [TX_PHY_DONE] -> Add TXEN Extension/1(IQ Done)
  S-R Latch2/1(Q) -> Register2/1
  Add TXEN Extension/1(RxSig Valid) -> Logical8/1
  Register2/1 -> RX_SIGS_INVALID/1
  Logical6/1 -> S-R Latch/2(R)
  Logical7/1 -> S-R Latch1/2(R)
  Logical8/1 -> S-R Latch2/2(R)
  [TX_FORCE_RESET] -> Logical6/2, Logical8/2, Logical7/2
  Logical5/1 -> Pkt Buf Sel/1(Sw Tx), Tx Gain/1(Sw Tx), PHY Mode Sel/1(Sw Tx)
  Pkt Buf Sel/1(Pkt Buf) -> [Tx_PKT_BUF_SEL]
  Tx Gain/1(Tx Gain A) -> [RC_IO_TX_GAIN_A]
  Tx Gain/2(Tx Gain B) -> [RC_IO_TX_GAIN_B]
  Tx Gain/3(Tx Gain C) -> [RC_IO_TX_GAIN_C]
  Tx Gain/4(Tx Gain D) -> [RC_IO_TX_GAIN_D]
  [MAC_IO_PHY_TX_ANT_MASK] -> Register4/1
  Register4/1 -> Register1/1
  Register1/1 -> [MAC_Tx_Ant_Mask]
  [regTx_Start_Direct] -> Logical5/2
  [regTx_Start_Indirect] -> Logical5/1
  [MAC_IO_PHY_TX_START] -> Pkt Buf Sel/2(Hw Tx), Tx Gain/2(Hw Tx), PHY Mode Sel/2(Hw Tx)
  [MAC_IO_PHY_TX_START] -> Register4/2
  [RC_IO_PHY_START] -> Logical/2
  Register3/1 -> PHY Start/1, Add MAC Extension/1(Tx Start)
  [regTx_Start_Direct] -> Logical/1
  [TX_PHY_DONE] -> Add MAC Extension/2(IQ Done)
  negedge/1(Q) -> [MAC_IO_PHY_TX_DONE], Simulation Stop/1(TX_DONE)
  Posedge2/1(Q) -> [MAC_IO_PHY_TX_STARTED]
  Add MAC Extension/1(Tx Active) -> negedge/1(D), Posedge2/1(D), Tx Active Debug Signal/1(Tx Active)
  Logical3/1 -> [Tx_PHY_Mode_11n_ac]
  Slice/1 -> [Tx_PHY_Mode_11ag]
  Slice1/1 -> [Tx_PHY_Mode_11n], Logical3/1
  Slice2/1 -> [Tx_PHY_Mode_11ac], Logical3/2
  PHY Mode Sel/1(PHY Mode) -> Slice/1, Slice1/1, Slice2/1, Gateway Out5/1
  Gateway Out5/1 -> Display/1
  Logical/1 -> Register3/1
  [TX_IQ_SAMP_CE] -> Register3/2
  [regTx_RC_RXEN_ENABLE] -> Posedge4/1(D)
  Posedge4/1(Q) -> Logical4/1
  Posedge5/1(Q) -> Logical4/2
  Posedge1/1(Q) -> S-R Latch/1(S), S-R Latch2/1(S), Logical7/1

== system wlan_phy_tx_pmd/HT Preamble Gen/S-R Latch1 ==
  S : Inport
  R : Inport  Port=2
  Constant1 : xbsIndex_r4/Constant  const=1  gui_display_data_type=Fixed-point  arith_type=Boolean  n_bits=1  bin_pt=0  preci_type=Single  exp_width=8  frac_width=24  explicit_period=off  period=1  equ=P=C  opselect=C  inp2=PCIN>>17  opr=+  inp1=P  carry=CIN  dbl_ovrd=off  block_type=constant
      settings: block_version=VER_STRING_GOES_HERE
  Convert1 : xbsIndex_r4/Convert  gui_display_data_type=Boolean  arith_type=Boolean  n_bits=1  bin_pt=0  float_type=Single  exp_bits=8  fraction_bits=24  quantization=Truncate  overflow=Wrap  en=off  latency=0  dbl_ovrd=off  pipeline=off  block_type=convert
  Convert2 : xbsIndex_r4/Convert  gui_display_data_type=Boolean  arith_type=Boolean  n_bits=1  bin_pt=0  float_type=Single  exp_bits=8  fraction_bits=24  quantization=Truncate  overflow=Wrap  en=off  latency=0  dbl_ovrd=off  pipeline=off  block_type=convert
  Register2 : xbsIndex_r4/Register  init=0  rst=on  en=on  dbl_ovrd=off  block_type=register
      settings: xl_area=[1 1 0 0 0 0 0]  block_version=VER_STRING_GOES_HERE
  Q : Outport
  wires:
  S/1 -> Convert2/1
  Register2/1 -> Q/1
  R/1 -> Convert1/1
  Constant1/1 -> Register2/1
  Convert1/1 -> Register2/2
  Convert2/1 -> Register2/3
